simulink model "offlineProcessingSathya"  (Simulink 8.0)
settings: Solver=ode45  StartTime=0.0  StopTime=10  RelTol=1e-3
undefined symbols (not defined in the file or in its folder): alphaMS, FS, magnitude, numSamplesPer20msFrame, psdMinBuf
libraries: dspstat3 x2, dspsigops x2, dspxfrm3 x1, dspsrcs4 x1, dspmathops x1, dspsnks4 x1
settings Model: Creator=Abhi  LastModifiedBy=Abhi
settings OptimizationCC: ExpressionDepthLimit=128
settings DebuggingCC: UnderspecifiedInitializationDetection=Simplified  SolverPrmCheckMsg=none  StateNameClashWarn=none
settings CodeAppCC: CustomSymbolStrType=$N$R$M_T
settings GRTTargetCC: CodeReplacementLibrary=C89/C90 (ANSI)

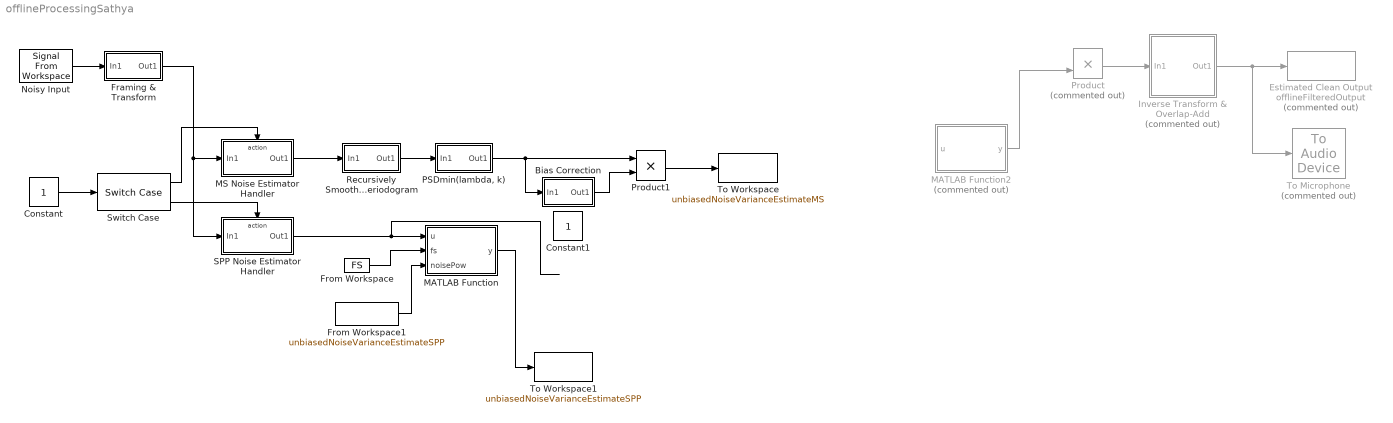
== system offlineProcessingSathya ==
  Bias Correction : Subsystem
  Constant : Constant
  Constant1 : Constant
  Estimated Clean Output : ToWorkspace  Commented=on  VariableName=offlineFilteredOutput  SaveFormat=Structure  SampleTime=-1
  Framing & Transform : Subsystem
  From Workspace : FromWorkspace  VariableName=FS  SampleTime=0
  From Workspace1 : FromWorkspace  VariableName=unbiasedNoiseVarianceEstimateSPP  SampleTime=0
  Inverse Transform & Overlap-Add : Subsystem  Commented=on
  MATLAB Function : MATLAB Function  TreatAsAtomicUnit=on
      settings: PermitHierarchicalResolution=ParametersOnly
  MATLAB Function2 : MATLAB Function  Commented=on  TreatAsAtomicUnit=on
      settings: PermitHierarchicalResolution=ParametersOnly
  MS Noise Estimator Handler : Subsystem  TreatAsAtomicUnit=on
  Noisy Input : dspsrcs4/Signal From Workspace  X=U  Ts=1/FS  nsamps=numSamplesPer20msFrame  OutputAfterFinalValue=Setting to zero  ignoreOrWarnInputAndFrameLengths=off
  "PSDmin(lambda, k)" : Subsystem
  Product : Product  Commented=on
  Product1 : Product
  Recursively Smoothed Periodogram : Subsystem
  SPP Noise Estimator Handler : Subsystem  TreatAsAtomicUnit=on
  Switch Case : SwitchCase  CaseConditions={1,2}  ShowDefaultCase=off
  To Microphone : dspsnks4/To Audio Device  Commented=on  deviceName=Default  inheritSampleRate=on  sampleRate=44100  deviceDatatype=Determine from input data type  autoBufferSize=on  bufferSize=4096  queueDuration=1.0
  To Workspace : ToWorkspace  VariableName=unbiasedNoiseVarianceEstimateMS  SaveFormat=Timeseries  SampleTime=-1
  To Workspace1 : ToWorkspace  VariableName=unbiasedNoiseVarianceEstimateSPP  SaveFormat=Timeseries  SampleTime=-1
  wires:
  Noisy Input/1 -> Framing & Transform/1(In1)
  Inverse Transform & Overlap-Add/1(Out1) -> To Microphone/1, Estimated Clean Output/1
  MATLAB Function2/1(y) -> Product/2
  Product/1 -> Inverse Transform & Overlap-Add/1(In1)
  Constant/1 -> Switch Case/1
  Switch Case/1 -> MS Noise Estimator Handler/Action
  Switch Case/2 -> SPP Noise Estimator Handler/Action
  MS Noise Estimator Handler/1(Out1) -> Recursively Smoothed Periodogram/1(In1)
  Recursively Smoothed Periodogram/1(Out1) -> "PSDmin(lambda, k)"/1(In1)
  "PSDmin(lambda, k)"/1(Out1) -> Bias Correction/1(In1), Product1/1
  Bias Correction/1(Out1) -> Product1/2
  Product1/1 -> To Workspace/1
  Framing & Transform/1(Out1) -> SPP Noise Estimator Handler/1(In1), MS Noise Estimator Handler/1(In1)
  From Workspace/1 -> MATLAB Function/2(fs)
  SPP Noise Estimator Handler/1(Out1) -> MATLAB Function/1(u)
  MATLAB Function/1(y) -> To Workspace1/1
  From Workspace1/1 -> MATLAB Function/3(noisePow)

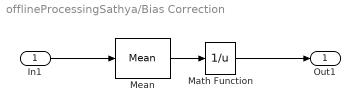
== system offlineProcessingSathya/Bias Correction ==
  In1 : Inport
  Math Function : Math  Operator=reciprocal  SaturateOnIntegerOverflow=on
  Mean : dspstat3/Mean  run=off  reset_popup=None  InputProcessing=Columns as channels (frame based)  directionMode=Each column  dimension=1  treatSBRowAsCol=on  roiEnable=off  roiType=Rectangles  roiPortion=Entire ROI  roiOutput=Individual statistics for each ROI  roiFlag=off  outputDataTypeStr=Inherit: Same as accumulator  outputLastDataTypeStr=Inherit: Same as accumulator  outputMin=[]  outputMax=[]  roundingMode=Floor  overflowMode=off
  Out1 : Outport
  wires:
  Math Function/1 -> Out1/1
  Mean/1 -> Math Function/1
  In1/1 -> Mean/1

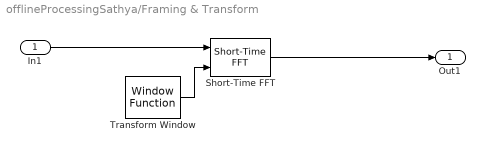
== system offlineProcessingSathya/Framing & Transform ==
  In1 : Inport
  Short-Time FFT : dspxfrm3/Short-Time FFT  W=numSamplesPer20msFrame  OvLap=overlapSamples  M=numSamplesPer20msFrame  TreatMby1Signals=One channel
  Transform Window : dspsigops/Window Function  winmode=Generate window  wintype=Hanning  sampmode=Discrete  samptime=1  N=numSamplesPer20msFrame  Rs=50  beta=10  winsamp=Symmetric  UserWindow=hamming  OptParams=off  UserParams={'symmetric'}  RowConvenienceOn=on  dataType=double  isSigned=on  wordLen=16  udDataType=sfix(16)  fracBitsMode=Best precision  numFracBits=15  roundingMode=Floor  overflowMode=off  numSidelobes=4  sidelobeLevel=-30
  Out1 : Outport
  wires:
  Short-Time FFT/1 -> Out1/1
  Transform Window/1 -> Short-Time FFT/2
  In1/1 -> Short-Time FFT/1

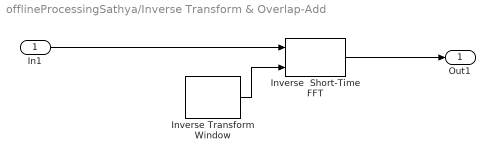
== system offlineProcessingSathya/Inverse Transform & Overlap-Add ==
  In1 : Inport
  Inverse Transform Window : Reference
  Inverse  Short-Time FFT : Reference
  Out1 : Outport
  wires:
  Inverse  Short-Time FFT/1 -> Out1/1
  Inverse Transform Window/1 -> Inverse  Short-Time FFT/2
  In1/1 -> Inverse  Short-Time FFT/1

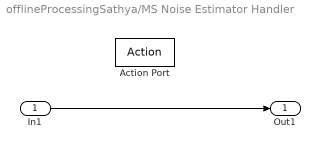
== system offlineProcessingSathya/MS Noise Estimator Handler ==
  In1 : Inport
  Action Port : ActionPort  ActionType=case
  Out1 : Outport
  wires:
  In1/1 -> Out1/1

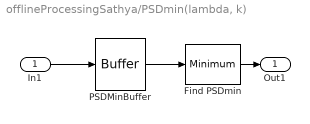
== system offlineProcessingSathya/PSDmin(lambda, k) ==
  In1 : Inport
  Find PSDmin : dspstat3/Minimum  fcn=Value  reset=None  InputProcessing=Columns as channels (frame based)  indexBase=One  operateOver=Each column  Dimension=1  colComp=on  operation=minimum  roiEnable=off  roiType=Rectangles  roiPortion=Entire ROI  roiOutput=Individual statistics for each ROI  roiFlag=off  roundingMode=Floor  overflowMode=off
  PSDMinBuffer : Buffer  N=psdMinBuf  V=psdMinBuf-1  TreatMby1Signals=One channel
  Out1 : Outport
  wires:
  PSDMinBuffer/1 -> Find PSDmin/1
  In1/1 -> PSDMinBuffer/1
  Find PSDmin/1 -> Out1/1

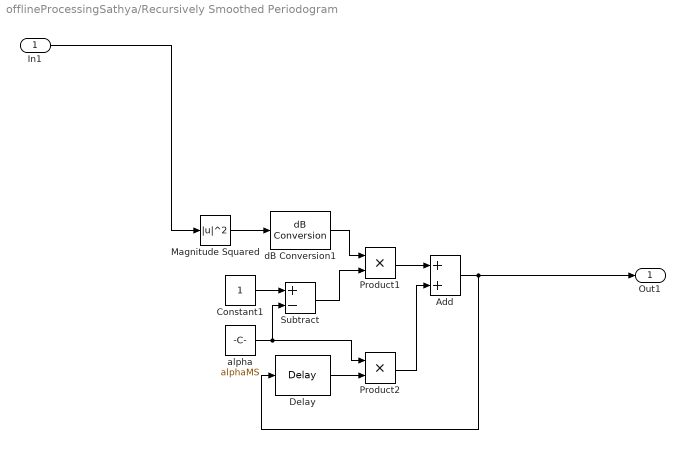
== system offlineProcessingSathya/Recursively Smoothed Periodogram ==
  In1 : Inport
  Add : Sum
  Constant1 : Constant
  Delay : dspsigops/Delay  InputProcessing=Columns as channels (frame based)  dly_unit=Frames  delay=1  ic_detail=off  dif_ic_for_ch=off  dif_ic_for_dly=off  ic=0  reset_popup=None
  Magnitude Squared : Math  Operator=magnitude^2  SaturateOnIntegerOverflow=on
  Product1 : Product
  Product2 : Product
  Subtract : Sum  Inputs=+-
  alpha : Constant  Value=alphaMS
  dB Conversion1 : dspmathops/dB Conversion  dBtype=dB  intype=Power  R=1  fuzz=off
  Out1 : Outport
  wires:
  Product2/1 -> Add/2
  In1/1 -> Magnitude Squared/1
  Add/1 -> Out1/1, Delay/1
  alpha/1 -> Product2/1, Subtract/2
  Product1/1 -> Add/1
  Constant1/1 -> Subtract/1
  dB Conversion1/1 -> Product1/1
  Delay/1 -> Product2/2
  Subtract/1 -> Product1/2
  Magnitude Squared/1 -> dB Conversion1/1

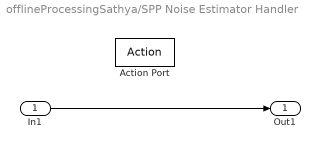
== system offlineProcessingSathya/SPP Noise Estimator Handler ==
  In1 : Inport
  Action Port : ActionPort  ActionType=case
  Out1 : Outport
  wires:
  In1/1 -> Out1/1

== matlab function MATLAB Function ==
  data: u input double; y output double; fs input double; noisePow input double
function y = fcn(u, fs, noisePow)
%#codegen

%% some constants
frLen   = 32e-3*fs;  % frame size % NOT CLEAR
fShift  = frLen/2;   % fShift size
nFrames = floor(length(u)/fShift)-1; % number of frames

anWin  = hanning(frLen,'periodic'); %analysis window

%% allocate some memory
noisePowMat = zeros(frLen/2+1,nFrames);


%% initialize
if noisePow == -1
    noisePow = init_noise_tracker_ideal_vad(u,frLen,frLen,fShift, anWin); % This function computes the initial noise PSD estimate. It is assumed that the first 5 time-frames are noise-only.
    y = noisePow;
    return;
end

%
PH1mean  = 0.5;
alphaPH1mean = 0.9;
alphaPSD = 0.8;

%constants for a posteriori SPP
q          = 0.5; % a priori probability of speech presence:
priorFact  = q./(1-q); % EQN (15) ???
% Fixing 15dB as the a priori SNR -> PAGE 6 Right (bottom)
xiOptDb    = 15; % optimal fixed a priori SNR for SPP estimation
xiOpt      = 10.^(xiOptDb./10);
logGLRFact = log(1./(1+xiOpt));
GLRexp     = xiOpt./(1+xiOpt);

% for indFr = 1:nFrames
%     indices       = (indFr-1)*fShift+1:(indFr-1)*fShift+frLen;
%     noisy_frame   = anWin.*noisy(indices);
%     noisyDftFrame = fft(noisy_frame,frLen); %512
%     noisyDftFrame = noisyDftFrame(1:frLen/2+1); %256
	
%     noisyPer = noisyDftFrame.*conj(noisyDftFrame); % <-(1)
    noisyPer = u.*conj(u); % <-(1)
    snrPost1 =  noisyPer./(noisePow);% a posteriori SNR based on old noise power estimate


    %% noise power estimation
	GLR     = priorFact .* exp(min(logGLRFact + GLRexp.*snrPost1,200));
	PH1     = GLR./(1+GLR); % a posteriori speech presence probability

	PH1mean  = alphaPH1mean * PH1mean + (1-alphaPH1mean) * PH1; % EQN (23)
	stuckInd = PH1mean > 0.99;                                  
	PH1(stuckInd) = min(PH1(stuckInd),0.99);                    % EQN (24)
	estimate =  PH1 .* noisePow + (1-PH1) .* noisyPer ; % noisyPer is obtained from DFT of windowed data over frame length -> (1) EQN (22)
	noisePow = alphaPSD *noisePow+(1-alphaPSD)*estimate;                                                                        % EQN (7)
        
% 	noisePowMat(:,indFr) = noisePow;
    y = noisePow;
% end
return





%%%%%%%%%%%%%%%%%%%%%%%%%%%%%%%%%%%%%%%%%%%%%%%%%%%%%%%%%%%%%%%%%%%%%%%%%%%%%%%%%%%%%%%


function   noise_psd_init =init_noise_tracker_ideal_vad(noisy,fr_size,fft_size,hop,sq_hann_window)
%%%%%%%%%%%%%%%%%%%%%%%%%%%%%%%%%%%%%%
%%%%This m-file computes an initial noise PSD estimate by means of a
%%%%Bartlett estimate.
%%%%Input parameters:   noisy:          noisy signal
%%%%                    fr_size:        frame size
%%%%                    fft_size:       fft size
%%%%                    hop:            hop size of frame
%%%%                    sq_hann_window: analysis window
%%%%Output parameters:  noise_psd_init: initial noise PSD estimate
%%%%
%%%%%%%%%%%%%%%%%%%%%%%%%%%%%%%%%%%%%%%%%%
%%%%%%%%%%%%%%%%%%%%%%Author: Richard C. Hendriks, 15/4/2010
%%%%%%%%%%%%%%%%%%%%%%%
%%%%%%%%%%%%%%%%%%%%%
 
for I=1:5
    noisy_frame=sq_hann_window.*noisy((I-1)*hop+1:(I-1)*hop+fr_size);
    noisy_dft_frame_matrix(:,I)=fft(noisy_frame,fft_size);
end
noise_psd_init=mean(abs(noisy_dft_frame_matrix(1:fr_size/2+1,1:end)).^2,2);%%%compute the initialisation of the noise tracking algorithms.
return

== matlab function MATLAB Function2 ==
  data: u input double; y output double
function y = calculateGain(u)
%#codegen

y = u;
